simulink model "untitled2"  (R2023b)
settings: Solver=FixedStepAuto  StartTime=0.0  StopTime=10.0  FixedStep=0.001  RelTol=1e-3
undefined symbols (not defined in the file): A, B, C, D, K, L, x0, x1, xi
settings Model: Creator=evdokiiagalkina  LastModifiedBy=evdokiiagalkina

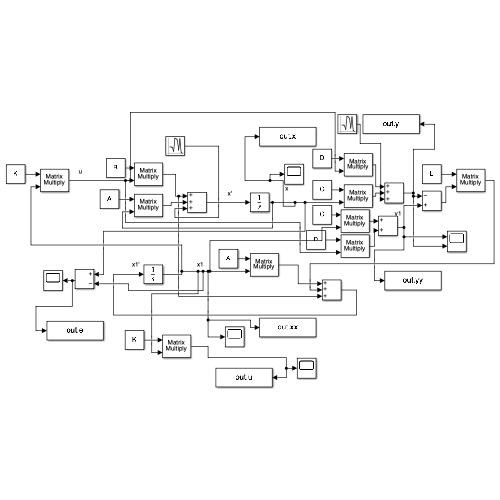
[thumbnail: Simulink's stored preview of the top-level diagram]
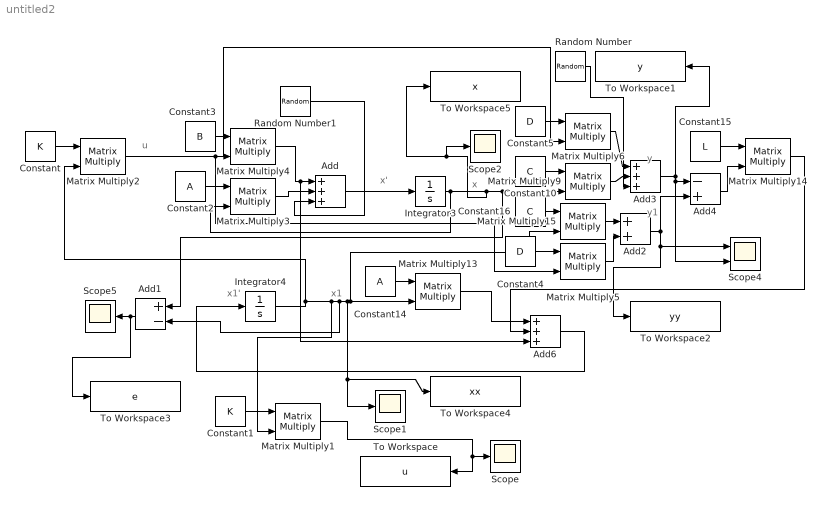
== system untitled2 ==
  note: x1
  note: x1'
  note: x
  note: u
  note: y1
  note: x'
  note: y
  Add : Sum  Inputs=+++
  Add1 : Sum  Inputs=+-
  Add2 : Sum
  Add3 : Sum  Inputs=+++
  Add4 : Sum  Inputs=-+
  Add6 : Sum  Inputs=+++
  Constant : Constant  Value=K  VectorParams1D=off
  Constant1 : Constant  Value=K  VectorParams1D=off
  Constant10 : Constant  Value=C  VectorParams1D=off
  Constant14 : Constant  Value=A  VectorParams1D=off
  Constant15 : Constant  Value=L  VectorParams1D=off
  Constant16 : Constant  Value=C  VectorParams1D=off
  Constant2 : Constant  Value=A  VectorParams1D=off
  Constant3 : Constant  Value=B  VectorParams1D=off
  Constant4 : Constant  Value=D  VectorParams1D=off
  Constant5 : Constant  Value=D  VectorParams1D=off
  Integrator3 : Integrator  InitialCondition=x0
  Integrator4 : Integrator  InitialCondition=x1
  Matrix Multiply{1..6,9,13..15} (10 alike) : Product  Multiplication=Matrix(*)
  Random Number : RandomNumber  Mean=xi  SampleTime=0.1
  Random Number1 : RandomNumber  Mean=fi  SampleTime=0.1
  Scope{,1..2,5} (4 alike) : Scope
  Scope4 : Scope  NumInputPorts=2
  To Workspace : ToWorkspace  VariableName=u  SaveFormat=Timeseries  SampleTime=-1
  To Workspace1 : ToWorkspace  VariableName=y  SaveFormat=Timeseries  SampleTime=-1
  To Workspace2 : ToWorkspace  VariableName=yy  SaveFormat=Timeseries  SampleTime=-1
  To Workspace3 : ToWorkspace  VariableName=e  SaveFormat=Timeseries  SampleTime=-1
  To Workspace4 : ToWorkspace  VariableName=xx  SaveFormat=Timeseries  SampleTime=-1
  To Workspace5 : ToWorkspace  VariableName=x  SaveFormat=Timeseries  SampleTime=-1
  wires:
  Constant10/1 -> Matrix Multiply9/1
  Constant14/1 -> Matrix Multiply13/1
  Integrator4/1 -> Matrix Multiply2/2, Add1/2, To Workspace4/1, Scope1/1, Matrix Multiply13/2, Matrix Multiply15/2, Matrix Multiply1/2
  Constant1/1 -> Matrix Multiply1/1
  Add1/1 -> To Workspace3/1, Scope5/1
  Constant/1 -> Matrix Multiply2/1
  Integrator3/1 -> Matrix Multiply3/2, To Workspace5/1, Scope2/1, Add1/1, Matrix Multiply9/2
  Constant3/1 -> Matrix Multiply4/1
  Matrix Multiply2/1 -> Matrix Multiply5/2, Matrix Multiply4/2, Matrix Multiply6/2
  Matrix Multiply4/1 -> Add6/3, Add/1
  Constant2/1 -> Matrix Multiply3/1
  Add6/1 -> Integrator4/1
  Constant15/1 -> Matrix Multiply14/1
  Matrix Multiply14/1 -> Add6/2
  Add4/1 -> Matrix Multiply14/2
  Matrix Multiply1/1 -> To Workspace/1, Scope/1
  Matrix Multiply13/1 -> Add6/1
  Matrix Multiply3/1 -> Add/2
  Add/1 -> Integrator3/1
  Constant16/1 -> Matrix Multiply15/1
  Matrix Multiply15/1 -> Add2/1
  Add2/1 -> To Workspace2/1, Scope4/1, Add4/2
  Matrix Multiply5/1 -> Add2/2
  Constant4/1 -> Matrix Multiply5/1
  Add3/1 -> To Workspace1/1, Scope4/2, Add4/1
  Matrix Multiply9/1 -> Add3/2
  Matrix Multiply6/1 -> Add3/1
  Constant5/1 -> Matrix Multiply6/1
  Random Number/1 -> Add3/3
  Random Number1/1 -> Add/3
